simulink model "minseg_nonlinear"  (R2024a)
settings: Solver=VariableStepAuto  StartTime=0.0  StopTime=tsim  RelTol=1e-3
values from neighbouring files (symbols this model uses):
  KLQR = lqr(A, B, Q, R)    [sim_minseg.m]
  ref = [0;0;0;0]    [sim_minseg.m]
  xs = [0;0;10/180*pi;0]    [sim_minseg.m]
settings Model: Creator=Meenakshi Mahagaokar  LastModifiedBy=Meenakshi Mahagaokar
settings DataIOCC: SaveOutput=off  DSMLogging=off  SaveTime=off  ReturnWorkspaceOutputs=off

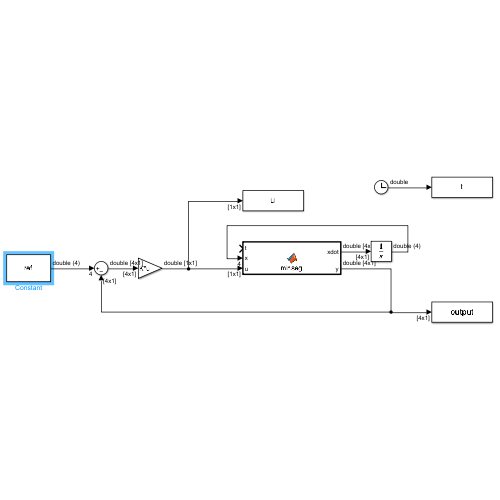
[thumbnail: Simulink's stored preview of the top-level diagram]
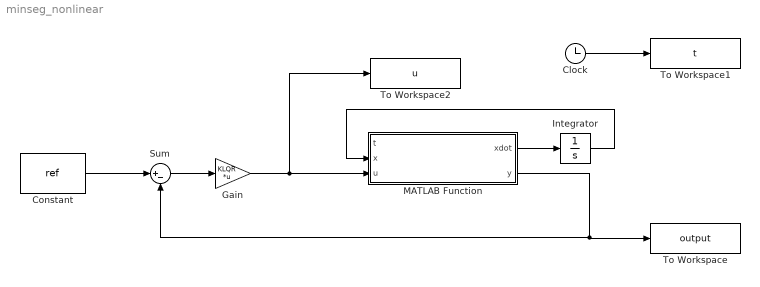
== system minseg_nonlinear ==
  Clock : Clock
  Constant : Constant  Value=ref
  Gain : Gain  Gain=KLQR  Multiplication=Matrix(K*u)
  Integrator : Integrator  InitialCondition=xs
  MATLAB Function : MATLAB Function  TreatAsAtomicUnit=on
  Sum : Sum  Inputs=|+-
  To Workspace : ToWorkspace  VariableName=output  SampleTime=-1
      settings: Save2DSignal=2-D array (concatenate along first dimension)
  To Workspace1 : ToWorkspace  VariableName=t  SampleTime=-1
      settings: Save2DSignal=2-D array (concatenate along first dimension)
  To Workspace2 : ToWorkspace  VariableName=u  SampleTime=-1
      settings: Save2DSignal=2-D array (concatenate along first dimension)
  wires:
  Sum/1 -> Gain/1
  Integrator/1 -> MATLAB Function/2(x)
  MATLAB Function/1(xdot) -> Integrator/1
  MATLAB Function/2(y) -> To Workspace/1, Sum/2
  Clock/1 -> To Workspace1/1
  Constant/1 -> Sum/1
  Gain/1 -> To Workspace2/1, MATLAB Function/3(u)

== matlab function minseg_nonlinear/MATLAB Function ==
  data: t input; x input; xdot output; u input; y output
function [xdot,y] = minseg(t, x, u)

xdot = minseg(t, x, u);
y = [x(1);
    x(2);
    x(3);
    x(4)];
